simulink model "MotorInteraction"  (R2024a)
settings: Solver=VariableStepAuto  StartTime=0.0  StopTime=10.0  RelTol=1e-3
model workspace (MATLAB code in the model file):
  | whangle = Simulink.Parameter(0.0);
  | whangle.Unit = 'rad';
  | 
  | WheelParams;
undefined symbols (not defined in the file): wheel_distance, wheel_lineardrivetraction, wheel_radius, wheel_staticdrivetraction, wheel_strafetraction, wheel_subwheels
settings Model: ParameterArgumentNames=whangle  Creator=Marij  LastModifiedBy=Marij
settings OptimizationCC: UseDivisionForNetSlopeComputation=on
settings ModelReferenceCC: ModelReferenceMinAlgLoopOccurrences=on

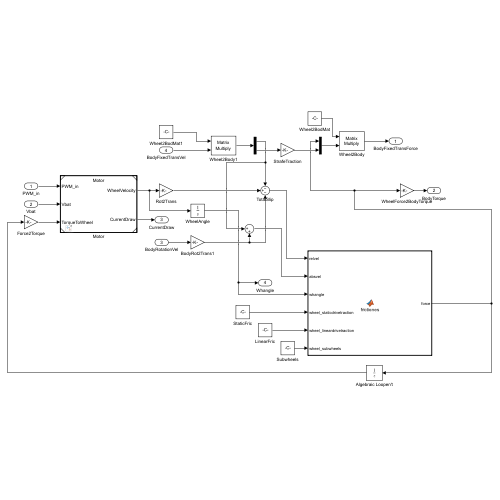
[thumbnail: Simulink's stored preview of the top-level diagram]
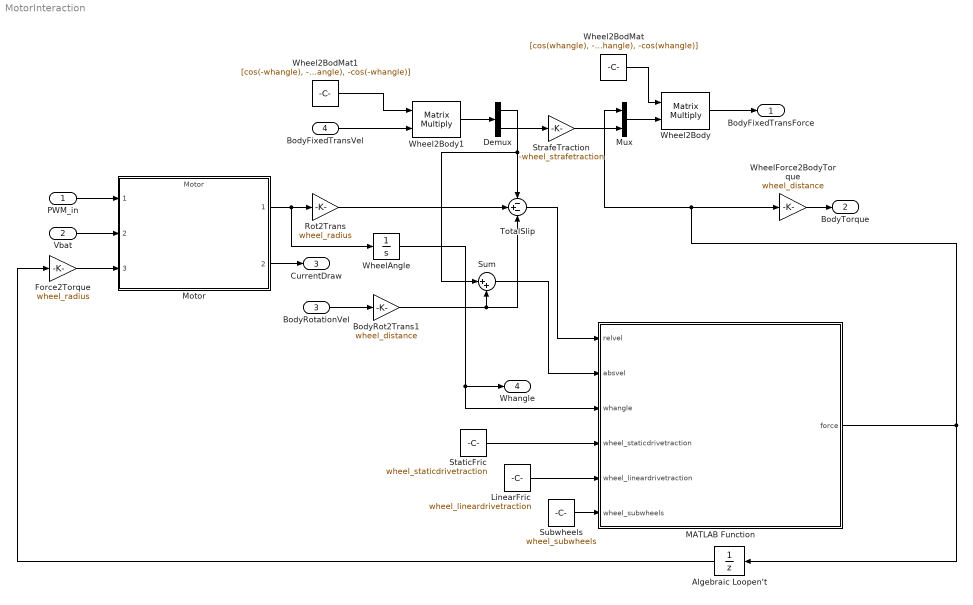
== system MotorInteraction ==
  PWM_in : Inport
  Vbat : Inport  Port=2
  BodyRotationVel : Inport  Port=3  Unit=rad/s
  BodyFixedTransVel : Inport  Port=4  Unit=m/s  PortDimensions=2
  Algebraic Loopen't : UnitDelay  SampleTime=-1  HasFrameUpgradeWarning=on
  BodyRot2Trans1 : Gain  Gain=wheel_distance
  Demux : Demux  Outputs=2
  Force2Torque : Gain  Gain=wheel_radius
  LinearFric : Constant  Value=wheel_lineardrivetraction
  MATLAB Function : MATLAB Function  TreatAsAtomicUnit=on
  Motor : ModelReference  ModelNameDialog=Motor.slx  SimulationMode=Normal  ModelReferenceVersion=1.22
  Mux : Mux  Inputs=2
  Rot2Trans : Gain  Gain=wheel_radius
  StaticFric : Constant  Value=wheel_staticdrivetraction
  StrafeTraction : Gain  Gain=-wheel_strafetraction
  Subwheels : Constant  Value=wheel_subwheels
  Sum : Sum  Inputs=|++
  TotalSlip : Sum  Inputs=-+-
  Wheel2BodMat : Constant  Value=[cos(whangle), -sin(whangle); sin(whangle), -cos(whangle)]  VectorParams1D=off
  Wheel2BodMat1 : Constant  Value=[cos(-whangle), -sin(-whangle); sin(-whangle), -cos(-whangle)]  VectorParams1D=off
  Wheel2Body : Product  Multiplication=Matrix(*)
  Wheel2Body1 : Product  Multiplication=Matrix(*)
  WheelAngle : Integrator
  WheelForce2BodyTorque : Gain  Gain=wheel_distance
  BodyFixedTransForce : Outport  Unit=N  PortDimensions=2
  BodyTorque : Outport  Port=2  Unit=N*m
  CurrentDraw : Outport  Port=3  Unit=A  PortDimensions=1
  Whangle : Outport  Port=4
  wires:
  PWM_in/1 -> Motor/1
  Vbat/1 -> Motor/2
  Motor/1 -> WheelAngle/1, Rot2Trans/1
  Force2Torque/1 -> Motor/3
  Rot2Trans/1 -> TotalSlip/2
  Wheel2BodMat/1 -> Wheel2Body/1
  Wheel2Body/1 -> BodyFixedTransForce/1
  Mux/1 -> Wheel2Body/2
  TotalSlip/1 -> MATLAB Function/1(relvel)
  Demux/2 -> StrafeTraction/1
  Demux/1 -> Sum/1, TotalSlip/1
  StrafeTraction/1 -> Mux/2
  WheelForce2BodyTorque/1 -> BodyTorque/1
  BodyRotationVel/1 -> BodyRot2Trans1/1
  BodyRot2Trans1/1 -> Sum/2, TotalSlip/3
  Motor/2 -> CurrentDraw/1
  Sum/1 -> MATLAB Function/2(absvel)
  WheelAngle/1 -> Whangle/1, MATLAB Function/3(whangle)
  Algebraic Loopen't/1 -> Force2Torque/1
  StaticFric/1 -> MATLAB Function/4(wheel_staticdrivetraction)
  LinearFric/1 -> MATLAB Function/5(wheel_lineardrivetraction)
  Subwheels/1 -> MATLAB Function/6(wheel_subwheels)
  BodyFixedTransVel/1 -> Wheel2Body1/2
  Wheel2Body1/1 -> Demux/1
  Wheel2BodMat1/1 -> Wheel2Body1/1
  MATLAB Function/1(force) -> WheelForce2BodyTorque/1, Mux/1, Algebraic Loopen't/1

== matlab function MotorInteraction/MATLAB Function ==
  data: relvel input; force output; absvel input; whangle input; wheel_staticdrivetraction input; wheel_lineardrivetraction input; wheel_subwheels input
function force = frictiones(relvel, absvel, whangle, wheel_staticdrivetraction, wheel_lineardrivetraction, wheel_subwheels)
force = drivetraction_model(relvel, absvel, whangle, wheel_staticdrivetraction, wheel_lineardrivetraction, wheel_subwheels);
% force = drivetraction_linear(relvel, absvel, whangle, wheel_staticdrivetraction, wheel_lineardrivetraction, wheel_subwheels);
end
